simulink model "Dire_PID_controller"  (R2018a)
settings: Solver=FixedStepAuto  StartTime=0.0  StopTime=600  FixedStep=0.24  RelTol=1e-3
settings Model: Creator=热水器设计小微_E  LastModifiedBy=热水器设计小微_E

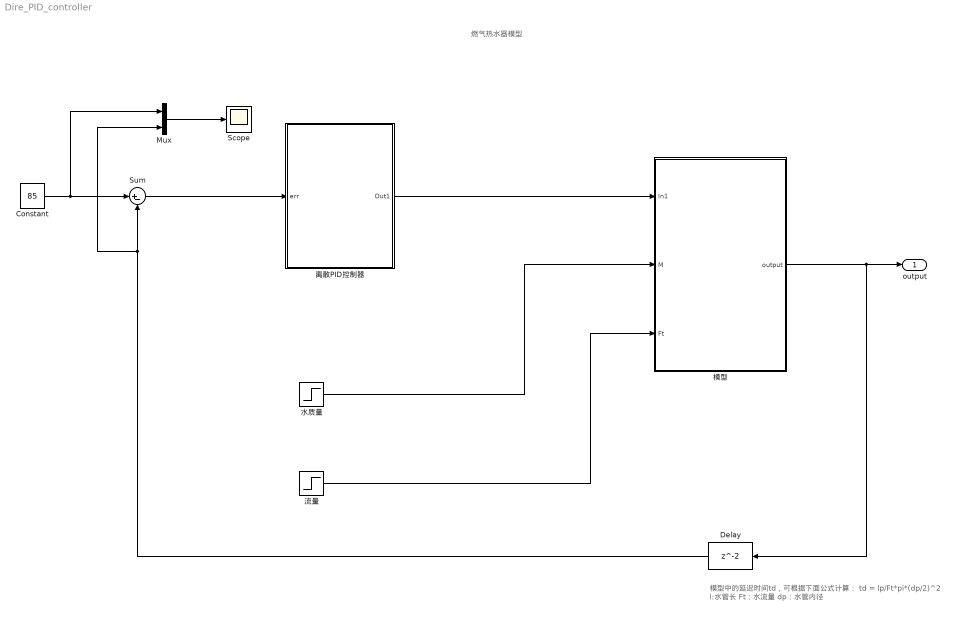
== system Dire_PID_controller ==
  note: 模型中的延迟时间td，可根据下面公式计算：
      |   td = lp/Ft*pi*(dp/2)^2
      | l:水管长
      | Ft：水流量
      | dp：水管内径
  note: 燃气热水器模型
  Constant : Constant  Value=85
  Delay : Delay
  Mux : Mux  Inputs=2
  Scope : Scope
  Sum : Sum  Inputs=|+-
  模型 : Subsystem  mask{Ts=0.0001, Q=10, C=6.8, y=0.5}
      mask prompts: Ts "采样时间"; Q "燃烧值"; C "比热容"; y "热效率"
  水质量 : Step  Before=5  After=40  SampleTime=0
  流量 : Step  Before=5  After=2  SampleTime=0
  离散PID控制器 : Subsystem  mask{Kp=2500, Ki=500, Kd=400, N=100, Ts=0.24}
      mask prompts: Kp "比例增益"; Ki "积分增益"; Kd "微分增益"; N "滤波系数"; Ts "采样时间"
  output : Outport
  wires:
  离散PID控制器/1(Out1) -> 模型/1(In1)
  模型/1(output) -> Delay/1, output/1
  水质量/1 -> 模型/2(M)
  流量/1 -> 模型/3(Ft)
  Sum/1 -> 离散PID控制器/1(err)
  Constant/1 -> Mux/1, Sum/1
  Mux/1 -> Scope/1
  Delay/1 -> Mux/2, Sum/2

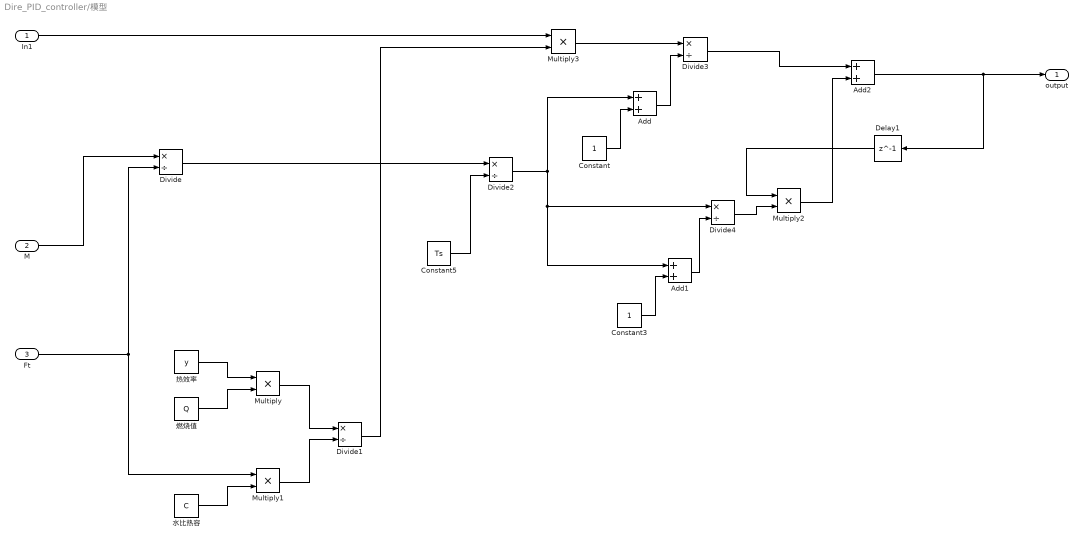
== system Dire_PID_controller/模型 ==
  In1 : Inport
  M : Inport  Port=2
  Ft : Inport  Port=3
  Add : Sum
  Add1 : Sum
  Add2 : Sum
  Constant : Constant
  Constant3 : Constant
  Constant5 : Constant  Value=Ts
  Delay1 : Delay  DelayLength=1
  Divide{,1..4} (5 alike) : Product  Inputs=*/
  Multiply{,1..3} (4 alike) : Product
  水比热容 : Constant  Value=C
  热效率 : Constant  Value=y
  燃烧值 : Constant  Value=Q
  output : Outport
  wires:
  热效率/1 -> Multiply/1
  Ft/1 -> Multiply1/1, Divide/2
  Multiply1/1 -> Divide1/2
  燃烧值/1 -> Multiply/2
  Divide3/1 -> Add2/1
  Constant/1 -> Add/2
  Add/1 -> Divide3/2
  Divide/1 -> Divide2/1
  Divide1/1 -> Multiply3/2
  Add2/1 -> output/1, Delay1/1
  Divide2/1 -> Add1/1, Divide4/1, Add/1
  Delay1/1 -> Multiply2/1
  Multiply2/1 -> Add2/2
  Multiply3/1 -> Divide3/1
  In1/1 -> Multiply3/1
  Constant5/1 -> Divide2/2
  Divide4/1 -> Multiply2/2
  Add1/1 -> Divide4/2
  Constant3/1 -> Add1/2
  Multiply/1 -> Divide1/1
  M/1 -> Divide/1
  水比热容/1 -> Multiply1/2

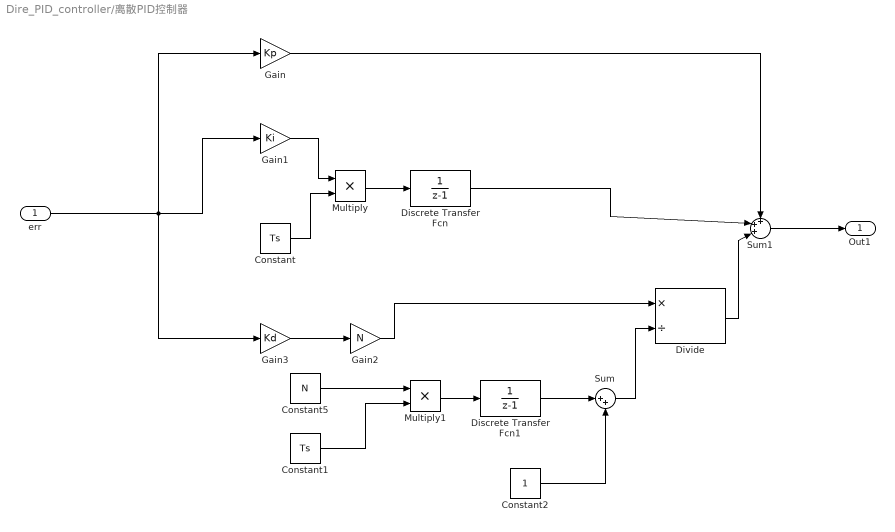
== system Dire_PID_controller/离散PID控制器 ==
  err : Inport
  Constant : Constant  Value=Ts
  Constant1 : Constant  Value=Ts
  Constant2 : Constant
  Constant5 : Constant  Value=N
  Discrete Transfer Fcn : DiscreteTransferFcn  Denominator=[1 -1]
  Discrete Transfer Fcn1 : DiscreteTransferFcn  Denominator=[1 -1]
  Divide : Product  Inputs=*/
  Gain : Gain  Gain=Kp
  Gain1 : Gain  Gain=Ki
  Gain2 : Gain  Gain=N
  Gain3 : Gain  Gain=Kd
  Multiply : Product
  Multiply1 : Product
  Sum : Sum  Inputs=|++
  Sum1 : Sum  Inputs=+++|
  Out1 : Outport
  wires:
  Gain2/1 -> Divide/1
  Sum/1 -> Divide/2
  Constant1/1 -> Multiply1/2
  Discrete Transfer Fcn/1 -> Sum1/2
  Multiply/1 -> Discrete Transfer Fcn/1
  Gain3/1 -> Gain2/1
  Discrete Transfer Fcn1/1 -> Sum/1
  Multiply1/1 -> Discrete Transfer Fcn1/1
  Gain/1 -> Sum1/1
  Constant2/1 -> Sum/2
  Constant/1 -> Multiply/2
  Divide/1 -> Sum1/3
  Gain1/1 -> Multiply/1
  Sum1/1 -> Out1/1
  err/1 -> Gain/1, Gain1/1, Gain3/1
  Constant5/1 -> Multiply1/1
